simulink model "app3_simulink"  (R2015b)
settings: Solver=VariableStepAuto  StartTime=0.0  StopTime=10.0  RelTol=1e-3
values from neighbouring files (symbols this model uses):
  A = [0 0 1 0; 0 0 0 1; 0 0 0 0; 0 0 0 0]    [app_code.m]
  B = [0; 0; 0; 1]    [app_code.m]
  C = [0 1 0 0; 1 0 0 0]    [app_code.m]
  D = [0; 0]    [app_code.m]
  g = -5    [app_code.m]
  init_cond = [x0; y0; vx0; vy0]    [app_code.m]
settings Model: Creator=pgarneau  LastModifiedBy=pgarneau

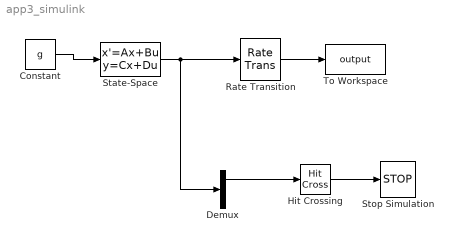
== system app3_simulink ==
  Constant : Constant  Value=g
  Demux : Demux  Outputs=2
  Hit Crossing : HitCross  HitCrossingOffset=bottom_out  HitCrossingDirection=falling
  Rate Transition : RateTransition  OutPortSampleTime=1/24
  State-Space : StateSpace  A=A  B=B  C=C  D=D  X0=init_cond
  Stop Simulation : Stop
  To Workspace : ToWorkspace  VariableName=output  SaveFormat=Timeseries  SampleTime=-1
  wires:
  Constant/1 -> State-Space/1
  Demux/1 -> Hit Crossing/1
  Hit Crossing/1 -> Stop Simulation/1
  State-Space/1 -> Rate Transition/1, Demux/1
  Rate Transition/1 -> To Workspace/1
